simulink model "Glucose_Insulin_Dynamics"  (R2014b)
settings: Solver=ode45  StartTime=0.0  StopTime=0  FixedStep=.01  MaxStep=.01  RelTol=1e-6
settings Model: Creator=Elise  LastModifiedBy=Eric
settings DataIOCC: FinalStateName=steady_state_glucose_insulin  LimitDataPoints=off  SaveFinalState=on  SaveCompleteFinalSimState=on

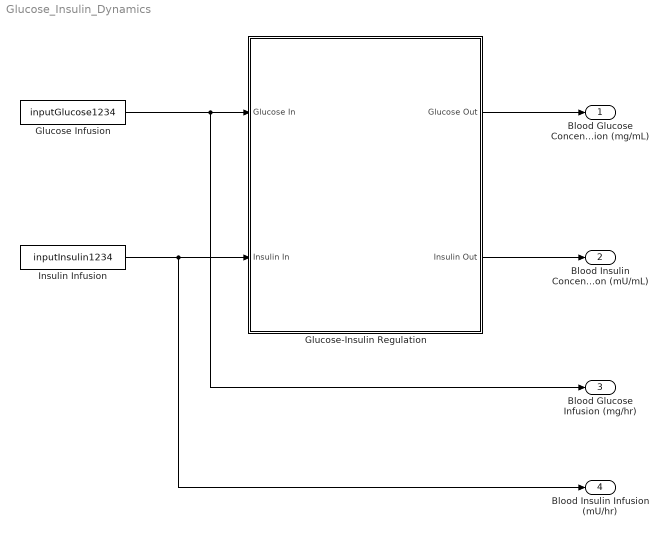
== system Glucose_Insulin_Dynamics ==
  Glucose Infusion : FromWorkspace  VariableName=inputGlucose1234  SampleTime=0  OutputAfterFinalValue=Setting to zero
  Glucose-Insulin Regulation : Subsystem
  Insulin Infusion : FromWorkspace  VariableName=inputInsulin1234  SampleTime=0  OutputAfterFinalValue=Setting to zero
  Blood Glucose Concentration (mg/mL) : Outport
  Blood Insulin Concentration (mU/mL) : Outport  Port=2
  Blood Glucose Infusion (mg/hr) : Outport  Port=3
  Blood Insulin Infusion (mU/hr) : Outport  Port=4
  wires:
  Glucose-Insulin Regulation/1(Glucose Out) -> Blood Glucose Concentration (mg/mL)/1
  Glucose-Insulin Regulation/2(Insulin Out) -> Blood Insulin Concentration (mU/mL)/1
  Glucose Infusion/1 -> Glucose-Insulin Regulation/1(Glucose In), Blood Glucose Infusion (mg/hr)/1
  Insulin Infusion/1 -> Blood Insulin Infusion (mU/hr)/1, Glucose-Insulin Regulation/2(Insulin In)

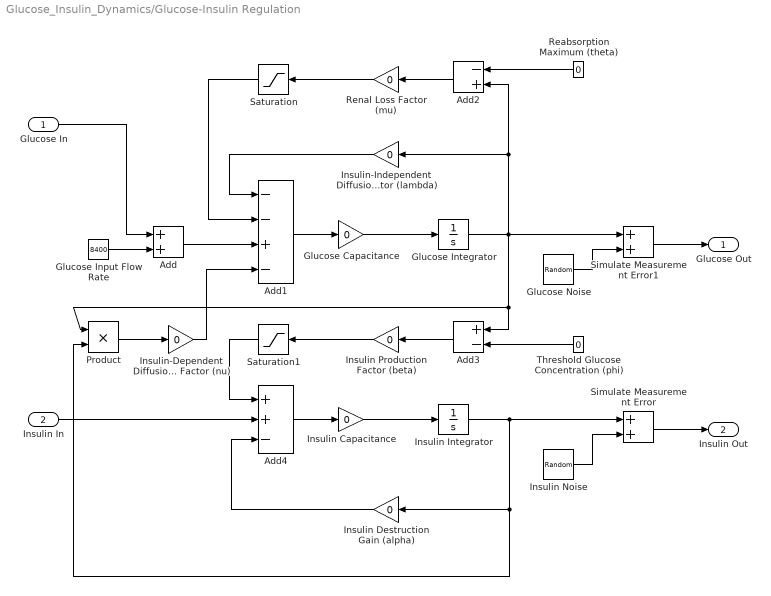
== system Glucose_Insulin_Dynamics/Glucose-Insulin Regulation ==
  Glucose In : Inport
  Insulin In : Inport  Port=2
  Add : Sum
  Add1 : Sum  Inputs=--+-
  Add2 : Sum  Inputs=-+
  Add3 : Sum  Inputs=+-
  Add4 : Sum  Inputs=++-
  Glucose Capacitance : Gain  Gain=0
  Glucose Input Flow Rate : Constant  Value=8400
  Glucose Integrator : Integrator
  Glucose Noise : RandomNumber  Variance=0  SampleTime=.01
  Insulin Capacitance : Gain  Gain=0
  Insulin Destruction Gain (alpha) : Gain  Gain=0
  Insulin Integrator : Integrator
  Insulin Noise : RandomNumber  Variance=0  SampleTime=.01
  Insulin Production Factor (beta) : Gain  Gain=0
  Insulin-Dependent Diffusion Factor (nu) : Gain  Gain=0
  Insulin-Independent Diffusion Factor (lambda) : Gain  Gain=0
  Product : Product
  Reabsorption Maximum (theta) : Constant  Value=0
  Renal Loss Factor (mu) : Gain  Gain=0
  Saturation : Saturate  UpperLimit=10000000  LowerLimit=0
  Saturation1 : Saturate  UpperLimit=10000000  LowerLimit=0
  Simulate Measurement Error : Sum
  Simulate Measurement Error1 : Sum
  Threshold Glucose Concentration (phi) : Constant  Value=0
  Glucose Out : Outport
  Insulin Out : Outport  Port=2
  wires:
  Glucose Input Flow Rate/1 -> Add/2
  Glucose In/1 -> Add/1
  Add/1 -> Add1/3
  Add1/1 -> Glucose Capacitance/1
  Glucose Capacitance/1 -> Glucose Integrator/1
  Insulin-Independent Diffusion Factor (lambda)/1 -> Add1/1
  Add2/1 -> Renal Loss Factor (mu)/1
  Reabsorption Maximum (theta)/1 -> Add2/1
  Renal Loss Factor (mu)/1 -> Saturation/1
  Saturation/1 -> Add1/2
  Threshold Glucose Concentration (phi)/1 -> Add3/2
  Add3/1 -> Insulin Production Factor (beta)/1
  Insulin Production Factor (beta)/1 -> Saturation1/1
  Saturation1/1 -> Add4/1
  Add4/1 -> Insulin Capacitance/1
  Insulin Capacitance/1 -> Insulin Integrator/1
  Product/1 -> Insulin-Dependent Diffusion Factor (nu)/1
  Insulin-Dependent Diffusion Factor (nu)/1 -> Add1/4
  Glucose Integrator/1 -> Simulate Measurement Error1/1, Add2/2, Insulin-Independent Diffusion Factor (lambda)/1, Add3/1, Product/1
  Insulin Integrator/1 -> Simulate Measurement Error/1, Product/2, Insulin Destruction Gain (alpha)/1
  Insulin Noise/1 -> Simulate Measurement Error/2
  Simulate Measurement Error/1 -> Insulin Out/1
  Glucose Noise/1 -> Simulate Measurement Error1/2
  Simulate Measurement Error1/1 -> Glucose Out/1
  Insulin Destruction Gain (alpha)/1 -> Add4/3
  Insulin In/1 -> Add4/2
